simulink model "TV_2017"  (R2016a)
settings: Solver=FixedStepAuto  StartTime=0.0  StopTime=inf  FixedStep=0.001  RelTol=1e-3
PreLoadFcn:
  | TV_2017_parameters
values from neighbouring files (symbols this model uses):
  battery_voltage = single(530)    [HIL_parameters.m]    (also in HIL_parameters_2018.m; TV_2017_parameters.m; TV_2017_parameters_VD.m)
  car_params = Simulink_Car_params    [HIL_parameters.m]    (also in HIL_parameters_2018.m; TV_2017_parameters.m; TV_2017_parameters_VD.m)
  i_Diff = 16    [HIL_parameters.m]    (also in HIL_parameters_2018.m; TV_2017_parameters.m)
  Kp = 1    [HIL_parameters.m]    (also in HIL_parameters_2018.m; TV_2017_parameters.m; TV_2017_parameters_VD.m)
  motor_data = struct    [HIL_parameters.m]    (also in HIL_parameters_2018.m; TV_2017_parameters.m)
  powerLimitControl = Simulink_el    [HIL_parameters.m]    (also in HIL_parameters_2018.m; TV_2017_parameters.m; TV_2017_parameters_VD.m)
  settings = Simulink_Settings    [HIL_parameters.m]    (also in HIL_parameters_2018.m; TV_2017_parameters.m; TV_2017_parameters_VD.m)
  SpdC_BCC = 0    [HIL_parameters.m]    (also in HIL_parameters_2018.m; TV_2017_parameters.m; TV_2017_parameters_VD.m)
  Speed_Neg_sat = -21    [HIL_parameters.m]    (also in HIL_parameters_2018.m; TV_2017_parameters.m; TV_2017_parameters_VD.m)
  Speed_Pos_sat = 21    [HIL_parameters.m]    (also in HIL_parameters_2018.m; TV_2017_parameters.m; TV_2017_parameters_VD.m)
  SteeringAngleFL = [-23.80 -22.65 -21.50 -20.34 -19.18 -18.03 -16.86 -15.70 -14.53 -13.35 -12.18 -10.99 -9.80 -8.61 -7.40 -6.19 -4.97 -3.75 -2.51 -1.26 0 1.27 2.56 3.85 5.17 6.50 7.84 9.21 10.59 12.00 13.42 14.88 16.36 17.87 19.41 20.99 22.61 24.26 25.97 27.73 29.54]    [CarSetupAnalysis2018.m]    (also in HIL_parameters_2018.m; TV_2017_parameters.m; TV_2017_parameters_VD.m = [-24.129 -22.950 -21.772 -20.593 -19.413 -18.232 -17.050 -15)
  SteeringAngleFR = [-29.54 -27.73 -25.97 -24.26 -22.61 -20.99 -19.41 -17.87 -16.36 -14.88 -13.42 -12.00 -10.59 -9.21 -7.84 -6.50 -5.17 -3.85 -2.56 -1.27 0 1.26 2.51 3.75 4.97 6.19 7.40 8.61 9.80 10.99 12.18 13.35 14.53 15.70 16.86 18.03 19.18 20.34 21.50 22.65 23.80]    [CarSetupAnalysis2018.m]    (also in HIL_parameters_2018.m; TV_2017_parameters.m; TV_2017_parameters_VD.m = [-29.3050 -27.5340 -25.8140 -24.1410 -22.5110 -20.9180 -19.3)
  SteeringWhAngle = [-105 -99.75 -94.5 -89.25 -84 -78.75 -73.5 -68.25 -63 -57.75 -52.5 -47.25 -42 -36.75 -31.5 -26.25 -21.0 -15.75 -10.5 -5.25 0.0 5.25 10.50 15.75 21.00 26.25 31.50 36.75 42.00 47.25 52.50 57.75  63.00 68.25 73.50 78.75 84.00 89.25 94.50 99.75 105.00]    [TV_2017_parameters_VD.m]
  Tn_n = 0    [HIL_parameters.m]    (also in HIL_parameters_2018.m; TV_2017_parameters.m; TV_2017_parameters_VD.m)
  tractionControl = Simulink_tc    [HIL_parameters.m]    (also in HIL_parameters_2018.m; IterativeTractionControlTuning.m; TV_2017_parameters.m; TV_2017_parameters_VD.m)
  yawMomentGenerator = struct    [HIL_parameters.m]    (also in HIL_parameters_2018.m = Simulink_yawRate2; TV_2017_parameters.m = Simulink_yawRate2)
  yawRateControl = Simulink_yawRate    [HIL_parameters.m]    (also in HIL_parameters_2018.m; TV_2017_parameters.m; TV_2017_parameters_VD.m)
undefined symbols (not defined in the file or in its folder): DiscIntNeverNeededParam, magnitude, speedEstimation, TC_Decr_Gas, TC_Derivative, TC_Incr_Gas, TC_On, TC_Relay_Off, TC_Relay_On
libraries: CarMaker4SL x350, simulink_extras x63, simulink x37, dspfdesign x2
(part 6 of 14)

== system TV_2017/CarMaker/Estimations/Fz_estimators/Fz_Estimation ==
  sensors : Inport
  1st_deriv : Subsystem
  2nd_deriv : Subsystem
  Bus Selector : BusSelector  OutputSignals=damper_rate_FL,damper_rate_FR,damper_rate_RL,damper_rate_RR
  Bus Selector1 : BusSelector  OutputSignals=FL,FR,RL,RR
  DamperRateLookup : Lookup_n-D  NumberOfTableDimensions=1  BreakpointsForDimension1=car_params.damper_table_breakpoint;  Table=car_params.damper_pull_push_values_front;  ExtrapMethod=Clip  UseLastTableValue=on  InternalRulePriority=Speed  RndMeth=Simplest  InputSameDT=on
  DamperRateLookup1 : Lookup_n-D  NumberOfTableDimensions=1  BreakpointsForDimension1=car_params.damper_table_breakpoint;  Table=car_params.damper_pull_push_values_front;  ExtrapMethod=Clip  UseLastTableValue=on  InternalRulePriority=Speed  RndMeth=Simplest  InputSameDT=on
  DamperRateLookup2 : Lookup_n-D  NumberOfTableDimensions=1  BreakpointsForDimension1=car_params.damper_table_breakpoint;  Table=car_params.damper_pull_push_values_rear;  ExtrapMethod=Clip  UseLastTableValue=on  InternalRulePriority=Speed  RndMeth=Simplest  InputSameDT=on
  DamperRateLookup3 : Lookup_n-D  NumberOfTableDimensions=1  BreakpointsForDimension1=car_params.damper_table_breakpoint;  Table=car_params.damper_pull_push_values_rear;  ExtrapMethod=Clip  UseLastTableValue=on  InternalRulePriority=Speed  RndMeth=Simplest  InputSameDT=on
  FZ_etsimate : Scope  NumInputPorts=4
  FzEstDamper : MATLAB Function  TreatAsAtomicUnit=on
  Scope2 : Scope  NumInputPorts=4
  Sum : Sum  Inputs=|++++
  Sum_FZ : Scope
  alfa_r_scope : Scope
  Fz_est : Outport
  alfa_r : Outport  Port=2
  wires:
  sensors/1 -> FzEstDamper/1(sensors), Bus Selector/1
  Bus Selector/1 -> DamperRateLookup/1  "<damper_rate_FL>"
  Bus Selector/2 -> DamperRateLookup1/1  "<damper_rate_FR>"
  Bus Selector/3 -> DamperRateLookup2/1  "<damper_rate_RL>"
  Bus Selector/4 -> DamperRateLookup3/1  "<damper_rate_RR>"
  FzEstDamper/2(alfa_r) -> alfa_r_scope/1, alfa_r/1
  Bus Selector1/2 -> Sum/3, FZ_etsimate/2  "<FR>"
  Bus Selector1/1 -> Sum/4, FZ_etsimate/1  "<FL>"
  Bus Selector1/3 -> Sum/2, FZ_etsimate/3  "<RL>"
  Bus Selector1/4 -> FZ_etsimate/4, Sum/1  "<RR>"
  FzEstDamper/1(Fz_damper_est) -> Bus Selector1/1, Fz_est/1
  DamperRateLookup1/1 -> Scope2/2, FzEstDamper/3(Fz_damp_FR)  "<FR>"
  DamperRateLookup/1 -> Scope2/1, FzEstDamper/2(Fz_damp_FL)  "<FL>"
  DamperRateLookup2/1 -> Scope2/3, FzEstDamper/4(Fz_damp_RL)  "<RL>"
  DamperRateLookup3/1 -> Scope2/4, FzEstDamper/5(Fz_damp_RR)  "<RR>"
  Sum/1 -> Sum_FZ/1

== system TV_2017/CarMaker/Estimations/Fz_estimators/Fz_Estimation_acceleration based ==
  sensors : Inport
  Bus Selector1 : BusSelector  OutputSignals=FL,FR,RL,RR
  Bus Selector2 : BusSelector  OutputSignals=Input_throttle,Input_brake,KERS_pos
  FZ_etsimate_acceleration : Scope  NumInputPorts=4
  Fz_acc_est : MATLAB Function  TreatAsAtomicUnit=on
  Lowpass Filter : dspfdesign/Lowpass Filter  FilterType=FIR  DesignForMinimumOrder=on  FilterOrder=50  PassbandFrequency=4  StopbandFrequency=15  PassbandRipple=0.1  StopbandAttenuation=80  InheritSampleRate=on  SampleRate=100  roundingMode=Floor  coeffsDataTypeStr=fixdt(1,16)  SimulateUsing=Interpreted execution
  Lowpass Filter1 : dspfdesign/Lowpass Filter  FilterType=FIR  DesignForMinimumOrder=on  FilterOrder=50  PassbandFrequency=4  StopbandFrequency=15  PassbandRipple=0.1  StopbandAttenuation=80  InheritSampleRate=on  SampleRate=100  roundingMode=Floor  coeffsDataTypeStr=fixdt(1,16)  SimulateUsing=Code generation
  alfa_r_acc : Scope  NumInputPorts=2
  alfa_r_acc_tps_bps_kers : Scope  NumInputPorts=4
  filtervsUnfilter : Scope  NumInputPorts=2
  "Fz_acc " : Outport
  "alfa_r_acc " : Outport  Port=2
  wires:
  sensors/1 -> Bus Selector2/1, Fz_acc_est/1(sensors)
  Bus Selector1/2 -> FZ_etsimate_acceleration/2  "<FR>"
  Bus Selector1/1 -> Lowpass Filter/1, filtervsUnfilter/2, FZ_etsimate_acceleration/1  "<FL>"
  Bus Selector1/3 -> FZ_etsimate_acceleration/3  "<RL>"
  Bus Selector1/4 -> FZ_etsimate_acceleration/4  "<RR>"
  Fz_acc_est/1(Fz_acc_est) -> "Fz_acc "/1, Bus Selector1/1
  Lowpass Filter/1 -> filtervsUnfilter/1
  Lowpass Filter1/1 -> alfa_r_acc/1
  Fz_acc_est/2(alfa_r_acc) -> alfa_r_acc_tps_bps_kers/1, "alfa_r_acc "/1, alfa_r_acc/2, Lowpass Filter1/1
  Bus Selector2/1 -> alfa_r_acc_tps_bps_kers/2  "<Input_throttle>"
  Bus Selector2/2 -> alfa_r_acc_tps_bps_kers/3  "<Input_brake>"
  Bus Selector2/3 -> alfa_r_acc_tps_bps_kers/4  "<KERS_pos>"

== system TV_2017/CarMaker/Estimations/Subsystem/SA calculation ==
  sensor : Inport
  Bus Selector2 : BusSelector  OutputSignals=steering_wheel_angle
  Degrees to Radians : simulink_extras/Transformations/Degrees to Radians
  Degrees to Radians1 : simulink_extras/Transformations/Degrees to Radians
  FL steer ang lookup deg : Lookup_n-D  NumberOfTableDimensions=1  BreakpointsForDimension1=SteeringAngleFL  Table=SteeringAngleFL  ExtrapMethod=Clip  UseLastTableValue=on  InternalRulePriority=Speed  RndMeth=Simplest  InputSameDT=on
  FR steer ang lookup deg : Lookup_n-D  NumberOfTableDimensions=1  BreakpointsForDimension1=SteeringAngleFR  Table=SteeringAngleFR  ExtrapMethod=Clip  UseLastTableValue=on  InternalRulePriority=Speed  RndMeth=Simplest  InputSameDT=on
  Radians to Degrees1 : simulink_extras/Transformations/Radians to Degrees
  Slip angle calc : MATLAB Function  Commented=on  TreatAsAtomicUnit=on
  Slip angle calc1 : MATLAB Function  TreatAsAtomicUnit=on
  SA : Outport
  wires:
  Radians to Degrees1/1 -> FL steer ang lookup deg/1, FR steer ang lookup deg/1
  Degrees to Radians1/1 -> Slip angle calc1/2(wheel_ang_right)
  Slip angle calc1/1(SA) -> SA/1
  FR steer ang lookup deg/1 -> Degrees to Radians1/1
  sensor/1 -> Slip angle calc1/3(sensor), Bus Selector2/1
  FL steer ang lookup deg/1 -> Degrees to Radians/1
  Bus Selector2/1 -> Radians to Degrees1/1  "<steering_wheel_angle>"
  Degrees to Radians/1 -> Slip angle calc1/1(wheel_ang_left)

== system TV_2017/CarMaker/Estimations/Subsystem/SR_Calculation ==
  v_x : Inport
  whl_v : Inport  Port=2
  sensorInput : Inport  Port=3
  Slip ratio : MATLAB Function  TreatAsAtomicUnit=on
  SR : Outport
  wires:
  v_x/1 -> Slip ratio/1(V_x)
  Slip ratio/1(SR) -> SR/1
  whl_v/1 -> Slip ratio/2(whl_v)
  sensorInput/1 -> Slip ratio/3(sensor)

== system TV_2017/CarMaker/Estimations/Subsystem/Slip_Detection ==
  sensor : Inport
  SR : Inport  Port=2
  Memory : Memory  InheritSampleTime=on
  Slip Detection : MATLAB Function  TreatAsAtomicUnit=on
  slip : Outport
  wires:
  Slip Detection/1(slip) -> Memory/1, slip/1
  SR/1 -> Slip Detection/1(SR)
  sensor/1 -> Slip Detection/2(sensors)
  Memory/1 -> Slip Detection/3(slip_prev)

== system TV_2017/CarMaker/IPG Vehicle3/Brake/CreateBus Vhcl.Wheel.PT ==
  In : Inport
  BusCreator1 : BusCreator  Inputs=20
  Demux1 : Demux  Outputs=20
  Out : Outport
  wires:
  Demux1/20 -> BusCreator1/20  "Vhcl Trq_DriveSrc_trg d3"
  Demux1/19 -> BusCreator1/19  "Vhcl Trq_DriveSrc_trg d2"
  Demux1/18 -> BusCreator1/18  "Vhcl Trq_DriveSrc_trg d1"
  Demux1/17 -> BusCreator1/17  "Vhcl Trq_DriveSrc_trg d0"
  Demux1/16 -> BusCreator1/16  "Vhcl Wheel RR WhlBearing"
  Demux1/15 -> BusCreator1/15  "Vhcl Wheel RR Trq_T2W"
  Demux1/14 -> BusCreator1/14  "Vhcl Wheel RR Trq_BrakeReg_trg"
  Demux1/13 -> BusCreator1/13  "Vhcl Wheel RR Trq_Brake"
  Demux1/12 -> BusCreator1/12  "Vhcl Wheel RL WhlBearing"
  Demux1/11 -> BusCreator1/11  "Vhcl Wheel RL Trq_T2W"
  Demux1/10 -> BusCreator1/10  "Vhcl Wheel RL Trq_BrakeReg_trg"
  Demux1/9 -> BusCreator1/9  "Vhcl Wheel RL Trq_Brake"
  Demux1/8 -> BusCreator1/8  "Vhcl Wheel FR WhlBearing"
  Demux1/7 -> BusCreator1/7  "Vhcl Wheel FR Trq_T2W"
  Demux1/6 -> BusCreator1/6  "Vhcl Wheel FR Trq_BrakeReg_trg"
  Demux1/5 -> BusCreator1/5  "Vhcl Wheel FR Trq_Brake"
  Demux1/4 -> BusCreator1/4  "Vhcl Wheel FL WhlBearing"
  Demux1/3 -> BusCreator1/3  "Vhcl Wheel FL Trq_T2W"
  Demux1/2 -> BusCreator1/2  "Vhcl Wheel FL Trq_BrakeReg_trg"
  Demux1/1 -> BusCreator1/1  "Vhcl Wheel FL Trq_Brake"
  BusCreator1/1 -> Out/1
  In/1 -> Demux1/1

== system TV_2017/CarMaker/IPG Vehicle3/CarAndTrailer/CarAndTrailerUpd ==
  Sync_In : Inport
  Vhcl.Steering : Inport  Port=2
  Vhcl.Motion : Inport  Port=3
  Vhcl.PoI : Inport  Port=4
  Vhcl.Wheel.FL : Inport  Port=5
  Vhcl.Wheel.FR : Inport  Port=6
  Vhcl.Wheel.RL : Inport  Port=7
  Vhcl.Wheel.RR : Inport  Port=8
  Car.Hitch.FrcTrq : Inport  Port=9
  Vhcl.Fr1A : Inport  Port=10
  CarAndTrailerUpd : S-Function  FunctionName=CM_Sfun  Parameters='CarAndTrUpd'  SFunctionDeploymentMode=off  EnableBusSupport=off
  CreateBus Brake.IF.In : Subsystem
  Sync_Out : Outport
  Brake.IF.In : Outport  Port=2
  wires:
  Vhcl.Fr1A/1 -> CarAndTrailerUpd/10  "user vehicle only"
  Vhcl.Steering/1 -> CarAndTrailerUpd/2
  Vhcl.Motion/1 -> CarAndTrailerUpd/3
  Vhcl.PoI/1 -> CarAndTrailerUpd/4
  Vhcl.Wheel.FL/1 -> CarAndTrailerUpd/5
  Vhcl.Wheel.FR/1 -> CarAndTrailerUpd/6
  Car.Hitch.FrcTrq/1 -> CarAndTrailerUpd/9
  Vhcl.Wheel.RR/1 -> CarAndTrailerUpd/8
  Vhcl.Wheel.RL/1 -> CarAndTrailerUpd/7
  CarAndTrailerUpd/2 -> CreateBus Brake.IF.In/1(In)
  CreateBus Brake.IF.In/1(Out) -> Brake.IF.In/1
  CarAndTrailerUpd/1 -> Sync_Out/1
  Sync_In/1 -> CarAndTrailerUpd/1

== system TV_2017/CarMaker/IPG Vehicle3/CarAndTrailer/Forces ==
  Sync_In : Inport
  TireFL_In : Inport  Port=2
  TireFR_In : Inport  Port=3
  TireRL_In : Inport  Port=4
  TireRR_In : Inport  Port=5
  lSpring : Inport  Port=6
  vDamp : Inport  Port=7
  lStabi : Inport  Port=8
  lBuf : Inport  Port=9
  External Suspension Forces : Subsystem
  Tires : Subsystem
  Vehicle Forces : Subsystem
  Sync_Out : Outport
  Car.Virtual : Outport  Port=2
  Car.Aero : Outport  Port=3
  Car.Load : Outport  Port=4
  TireFL_Out : Outport  Port=5
  TireFR_Out : Outport  Port=6
  TireRL_Out : Outport  Port=7
  TireRR_Out : Outport  Port=8
  FSpring : Outport  Port=9
  FDamp : Outport  Port=10
  FStabi : Outport  Port=11
  FBuf : Outport  Port=12
  wires:
  lBuf/1 -> External Suspension Forces/5(lBuf)
  lStabi/1 -> External Suspension Forces/4(lStabi)
  vDamp/1 -> External Suspension Forces/3(vDamp)
  Tires/4(TireRR_Out) -> TireRR_Out/1
  Tires/3(TireRL_Out) -> TireRL_Out/1
  Tires/2(TireFR_Out) -> TireFR_Out/1
  Tires/1(TireFL_Out) -> TireFL_Out/1
  TireRR_In/1 -> Tires/5(TireRR_In)
  TireRL_In/1 -> Tires/4(TireRL_In)
  TireFR_In/1 -> Tires/3(TireFR_In)
  TireFL_In/1 -> Tires/2(TireFL_In)
  External Suspension Forces/4(FBuf) -> FBuf/1
  Sync_In/1 -> External Suspension Forces/1(Sync_In), Tires/1(Sync_In), Vehicle Forces/1(Sync_In)
  Vehicle Forces/1(Sync_Out) -> Sync_Out/1
  Vehicle Forces/2(Car.Virtual) -> Car.Virtual/1
  Vehicle Forces/3(Car.Aero) -> Car.Aero/1
  Vehicle Forces/4(Car.Load) -> Car.Load/1
  lSpring/1 -> External Suspension Forces/2(lSpring)
  External Suspension Forces/2(FDamp) -> FDamp/1
  External Suspension Forces/3(FStabi) -> FStabi/1
  External Suspension Forces/1(FSpring) -> FSpring/1

== system TV_2017/CarMaker/IPG Vehicle3/CarAndTrailer/Kinematics ==
  Sync_In : Inport
  Steer.IF : Inport  Port=2
  Kinematics : S-Function  FunctionName=CM_Sfun  Parameters='Kinematics'  SFunctionDeploymentMode=off  EnableBusSupport=off
  Sync_Out : Outport
  TireFL_In : Outport  Port=2
  TireFR_In : Outport  Port=3
  TireRL_In : Outport  Port=4
  TireRR_In : Outport  Port=5
  lSpring : Outport  Port=6
  vDamp : Outport  Port=7
  lStabi : Outport  Port=8
  lBuf : Outport  Port=9
  wires:
  Kinematics/9 -> lBuf/1
  Kinematics/8 -> lStabi/1
  Kinematics/2 -> TireFL_In/1
  Kinematics/3 -> TireFR_In/1
  Kinematics/4 -> TireRL_In/1
  Kinematics/5 -> TireRR_In/1
  Kinematics/6 -> lSpring/1
  Kinematics/7 -> vDamp/1
  Sync_In/1 -> Kinematics/1
  Kinematics/1 -> Sync_Out/1
  Steer.IF/1 -> Kinematics/2

== system TV_2017/CarMaker/IPG Vehicle3/CarAndTrailer/Kinetics ==
  Sync_In : Inport
  Car.Virtual : Inport  Port=2
  Car.Aero : Inport  Port=3
  Car.Load : Inport  Port=4
  TireFL.Out : Inport  Port=5
  TireFR.Out : Inport  Port=6
  TireRL.Out : Inport  Port=7
  TireRR.Out : Inport  Port=8
  FSpring : Inport  Port=9
  FDamp : Inport  Port=10
  FStabi : Inport  Port=11
  FBuf : Inport  Port=12
  Bus Creator : BusCreator  Inputs=4
  Bus Creator1 : BusCreator  Inputs=12
  Bus Creator2 : BusCreator  Inputs=6
  Bus Creator3 : BusCreator  Inputs=6
  Bus Creator4 : BusCreator  Inputs=4
  Demux : Demux  Outputs=12
  Demux1 : Demux  Outputs=6
  Demux2 : Demux  Outputs=6
  Demux3 : Demux
  Demux4 : Demux
  Kinetics : S-Function  FunctionName=CM_Sfun  Parameters='Kinetics'  SFunctionDeploymentMode=off  EnableBusSupport=off
  Sync_Out : Outport
  Trailer.Load : Outport  Port=2
  Car.Hitch : Outport  Port=3
  Car.Fr1 : Outport  Port=4
  Car.Trq_T2W : Outport  Port=5
  WheelCarrier.Misc : Outport  Port=6
  wires:
  FBuf/1 -> Kinetics/12
  Sync_In/1 -> Kinetics/1
  Kinetics/1 -> Sync_Out/1
  Car.Aero/1 -> Kinetics/3
  Car.Virtual/1 -> Kinetics/2
  Bus Creator1/1 -> Trailer.Load/1
  Demux/1 -> Bus Creator1/1  "Trailer Load_0 mass"
  Demux/2 -> Bus Creator1/2  "Trailer Load_0 tx"
  Demux/3 -> Bus Creator1/3  "Trailer Load_0 ty"
  Demux/4 -> Bus Creator1/4  "Trailer Load_0 tz"
  Kinetics/2 -> Demux/1
  Demux/5 -> Bus Creator1/5  "Trailer Load_1 mass"
  Demux/6 -> Bus Creator1/6  "Trailer Load_1 tx"
  Demux/7 -> Bus Creator1/7  "Trailer Load_1 ty"
  Demux/8 -> Bus Creator1/8  "Trailer Load_1 tz"
  Demux/9 -> Bus Creator1/9  "Trailer Load_2 mass"
  Demux/10 -> Bus Creator1/10  "Trailer Load_2 tx"
  Demux/11 -> Bus Creator1/11  "Trailer Load_2 ty"
  Demux/12 -> Bus Creator1/12  "Trailer Load_2 tz"
  Demux1/1 -> Bus Creator2/1  "Car Hitch tx"
  Demux1/2 -> Bus Creator2/2  "Car Hitch ty"
  Demux1/3 -> Bus Creator2/3  "Car Hitch tz"
  Demux1/4 -> Bus Creator2/4  "Car Hitch vx"
  Demux1/5 -> Bus Creator2/5  "Car Hitch vy"
  Demux1/6 -> Bus Creator2/6  "Car Hitch vz"
  Kinetics/3 -> Demux1/1
  Bus Creator2/1 -> Car.Hitch/1
  Demux2/1 -> Bus Creator3/1  "Car Fr1 rx"
  Demux2/2 -> Bus Creator3/2  "Car Fr1 ry"
  Demux2/3 -> Bus Creator3/3  "Car Fr1 rz"
  Demux2/4 -> Bus Creator3/4  "Car Fr1 rvx"
  Demux2/5 -> Bus Creator3/5  "Car Fr1 rvy"
  Demux2/6 -> Bus Creator3/6  "Car Fr1 rvz"
  Bus Creator3/1 -> Car.Fr1/1
  Kinetics/4 -> Demux2/1
  Car.Load/1 -> Kinetics/4
  Demux3/1 -> Bus Creator4/1  "car Susp FL GenInert2"
  Demux3/2 -> Bus Creator4/2  "car Susp FR GenInert2"
  Demux3/3 -> Bus Creator4/3  "car Susp FL GenFrc2"
  Demux3/4 -> Bus Creator4/4  "car Susp FR GenFrc2"
  Bus Creator4/1 -> WheelCarrier.Misc/1
  Bus Creator/1 -> Car.Trq_T2W/1
  Demux4/4 -> Bus Creator/4  "Car Trq_T2WRR"
  Demux4/3 -> Bus Creator/3  "Car Trq_T2WRL"
  Demux4/2 -> Bus Creator/2  "Car Trq_T2WFR"
  Demux4/1 -> Bus Creator/1  "Car Trq_T2WFL"
  TireFL.Out/1 -> Kinetics/5
  TireFR.Out/1 -> Kinetics/6
  TireRL.Out/1 -> Kinetics/7
  TireRR.Out/1 -> Kinetics/8
  FSpring/1 -> Kinetics/9
  FDamp/1 -> Kinetics/10
  FStabi/1 -> Kinetics/11
  Kinetics/6 -> Demux3/1
  Kinetics/5 -> Demux4/1

== system TV_2017/CarMaker/IPG Vehicle3/CarAndTrailer/Steering ==
  note: When replacing the entire steering system,
      | be sure to add '-disablesteering' to the command line arguments
      | in the CarMaker Model Configuration block.
  Sync_In : Inport
  VhclCtrl.Steering : Inport  Port=2
  Bus Creator1 : BusCreator  Inputs=16
  Bus Creator2 : BusCreator  Inputs=5
  Demux : Demux  Outputs=21
  Steering : S-Function  FunctionName=CM_Sfun  Parameters='Steering'  SFunctionDeploymentMode=off  EnableBusSupport=off
  Terminator : Terminator
  Sync_Out : Outport
  Steer.IF : Outport  Port=2
  wires:
  Demux/21 -> Bus Creator2/5  "Steering IF R Inert"
  Demux/20 -> Bus Creator2/4  "Steering IF R Frc"
  Demux/19 -> Bus Creator2/3  "Steering IF L Inert"
  Demux/18 -> Bus Creator2/2  "Steering IF L Frc"
  Demux/17 -> Bus Creator2/1  "Steering IF SteerByTrq"
  Demux/16 -> Bus Creator1/16  "Steering IF R iSteer2q"
  Demux/15 -> Bus Creator1/15  "Steering IF R qpp"
  Demux/14 -> Bus Creator1/14  "Steering IF R qp"
  Demux/13 -> Bus Creator1/13  "Steering IF R q"
  Demux/12 -> Bus Creator1/12  "Steering IF L iSteer2q"
  Demux/11 -> Bus Creator1/11  "Steering IF L qpp"
  Demux/10 -> Bus Creator1/10  "Steering IF L qp"
  Demux/9 -> Bus Creator1/9  "Steering IF L q"
  Demux/8 -> Bus Creator1/8  "Steering IF AssistTrqPin"
  Demux/7 -> Bus Creator1/7  "Steering IF AssistTrqCol"
  Demux/6 -> Bus Creator1/6  "Steering IF AssistFrc"
  Demux/5 -> Bus Creator1/5  "Steering IF TrqStatic"
  Demux/4 -> Bus Creator1/4  "Steering IF Trq"
  Demux/3 -> Bus Creator1/3  "Steering IF AngAcc"
  Demux/2 -> Bus Creator1/2  "Steering IF AngVel"
  Demux/1 -> Bus Creator1/1  "Steering IF Ang"
  Bus Creator1/1 -> Steer.IF/1
  Steering/2 -> Demux/1
  Bus Creator2/1 -> Terminator/1  "Steer IF (in)"
  VhclCtrl.Steering/1 -> Steering/2
  Steering/1 -> Sync_Out/1
  Sync_In/1 -> Steering/1

== system TV_2017/CarMaker/IPG Vehicle3/CarAndTrailer/Trailer ==
  Sync_In : Inport
  Trailer.Load : Inport  Port=2
  Car.Hitch : Inport  Port=3
  Car.Fr1 : Inport  Port=4
  Car.Trq_T2W : Inport  Port=5
  WheelCarrier.Misc : Inport  Port=6
  CreateBus Car.Hitch.FrcTrq : Subsystem
  CreateBus Vhcl.Motion : Subsystem
  CreateBus Vhcl.PoI : Subsystem
  CreateBus Vhcl.Steering : Subsystem
  CreateBus Vhcl.Wheel.FL : Subsystem
  CreateBus Vhcl.Wheel.FR : Subsystem
  CreateBus Vhcl.Wheel.RL : Subsystem
  CreateBus Vhcl.Wheel.RR : Subsystem
  Trailer : S-Function  FunctionName=CM_Sfun  Parameters='Trailer'  SFunctionDeploymentMode=off  EnableBusSupport=off
  Sync_Out : Outport
  Vhcl.Steering : Outport  Port=2
  Vhcl.Motion : Outport  Port=3
  Vhcl.PoI : Outport  Port=4
  Vhcl.Wheel.FL : Outport  Port=5
  Vhcl.Wheel.FR : Outport  Port=6
  Vhcl.Wheel.RL : Outport  Port=7
  Vhcl.Wheel.RR : Outport  Port=8
  Car.Hitch.FrcTrq : Outport  Port=9
  wires:
  Trailer/2 -> CreateBus Vhcl.Steering/1(In1)
  CreateBus Vhcl.Steering/1(Out1) -> Vhcl.Steering/1  "Vhcl.Steering"
  Trailer/3 -> CreateBus Vhcl.Motion/1(In1)
  Trailer/4 -> CreateBus Vhcl.PoI/1(In1)
  Trailer/5 -> CreateBus Vhcl.Wheel.FL/1(In1)
  Trailer/6 -> CreateBus Vhcl.Wheel.FR/1(In1)
  Trailer/7 -> CreateBus Vhcl.Wheel.RL/1(In1)
  Trailer/9 -> CreateBus Car.Hitch.FrcTrq/1(In1)
  Trailer/8 -> CreateBus Vhcl.Wheel.RR/1(In1)
  CreateBus Vhcl.Wheel.RR/1(Out1) -> Vhcl.Wheel.RR/1  "Vhcl.Wheel.RR"
  CreateBus Vhcl.Wheel.RL/1(Out1) -> Vhcl.Wheel.RL/1  "Vhcl.Wheel.RL"
  CreateBus Vhcl.Wheel.FR/1(Out1) -> Vhcl.Wheel.FR/1  "Vhcl.Wheel.FR"
  CreateBus Vhcl.Wheel.FL/1(Out1) -> Vhcl.Wheel.FL/1  "Vhcl.Wheel.FL"
  CreateBus Vhcl.PoI/1(Out1) -> Vhcl.PoI/1  "Vhcl.PoI"
  CreateBus Vhcl.Motion/1(Out1) -> Vhcl.Motion/1  "Vhcl.Motion"
  Car.Trq_T2W/1 -> Trailer/5
  WheelCarrier.Misc/1 -> Trailer/6
  CreateBus Car.Hitch.FrcTrq/1(Out1) -> Car.Hitch.FrcTrq/1  "Car.Hitch.FrcTrq"
  Car.Fr1/1 -> Trailer/4
  Car.Hitch/1 -> Trailer/3
  Trailer.Load/1 -> Trailer/2
  Trailer/1 -> Sync_Out/1
  Sync_In/1 -> Trailer/1

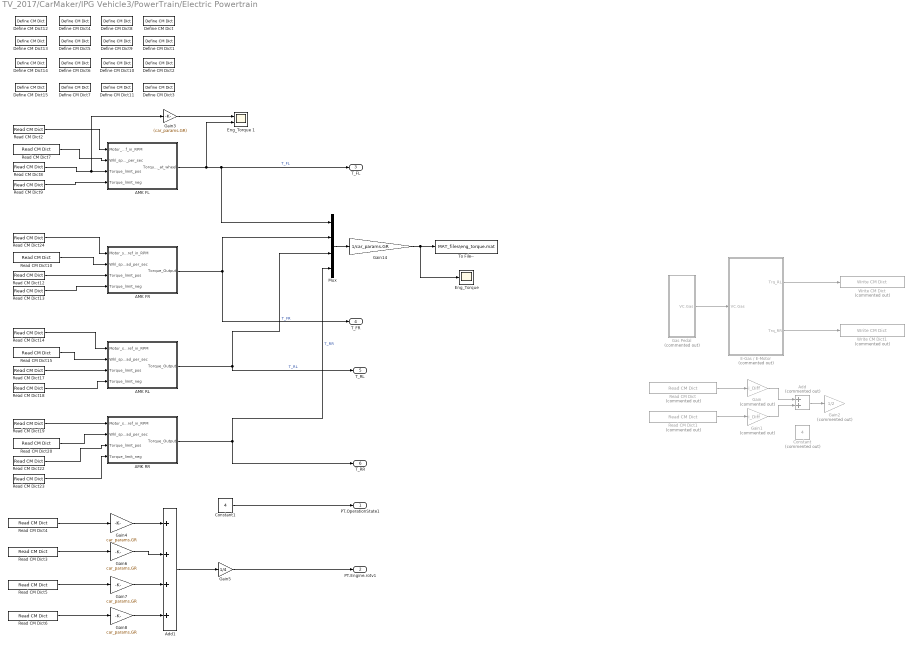
== system TV_2017/CarMaker/IPG Vehicle3/PowerTrain/Electric Powertrain ==
  AMK FL : Subsystem
  AMK FR : Subsystem
  AMK RL : Subsystem
  AMK RR : Subsystem
  Add : Sum  Commented=on
  Add1 : Sum  Inputs=++++
  Constant : Constant  Commented=on  Value=4
  Constant1 : Constant  Value=4
  Define CM Dict : CarMaker4SL/Define CM Dict  xname=T_req_RL  xmono=off  xtype=Double4  xdvaplace=None  xnstates=0  xfirststate=0  xinitial=0
  Define CM Dict1 : CarMaker4SL/Define CM Dict  xname=T_req_RR  xmono=off  xtype=Double4  xdvaplace=None  xnstates=0  xfirststate=0  xinitial=0
  Define CM Dict10 : CarMaker4SL/Define CM Dict  xname=Tlim_neg_RL  xmono=off  xtype=Double4  xdvaplace=None  xnstates=0  xfirststate=0  xinitial=0
  Define CM Dict11 : CarMaker4SL/Define CM Dict  xname=Tlim_neg_RR  xmono=off  xtype=Double4  xdvaplace=None  xnstates=0  xfirststate=0  xinitial=0
  Define CM Dict12 : CarMaker4SL/Define CM Dict  xname=w_set_FL  xmono=off  xtype=Double4  xdvaplace=None  xnstates=0  xfirststate=0  xinitial=0
  Define CM Dict13 : CarMaker4SL/Define CM Dict  xname=w_set_FR  xmono=off  xtype=Double4  xdvaplace=None  xnstates=0  xfirststate=0  xinitial=0
  Define CM Dict14 : CarMaker4SL/Define CM Dict  xname=w_set_RL  xmono=off  xtype=Double4  xdvaplace=None  xnstates=0  xfirststate=0  xinitial=0
  Define CM Dict15 : CarMaker4SL/Define CM Dict  xname=w_set_RR  xmono=off  xtype=Double4  xdvaplace=None  xnstates=0  xfirststate=0  xinitial=0
  Define CM Dict2 : CarMaker4SL/Define CM Dict  xname=T_req_FL  xmono=off  xtype=Double4  xdvaplace=None  xnstates=0  xfirststate=0  xinitial=0
  Define CM Dict3 : CarMaker4SL/Define CM Dict  xname=T_req_FR  xmono=off  xtype=Double4  xdvaplace=None  xnstates=0  xfirststate=0  xinitial=0
  Define CM Dict4 : CarMaker4SL/Define CM Dict  xname=Tlim_pos_FL  xmono=off  xtype=Double4  xdvaplace=None  xnstates=0  xfirststate=0  xinitial=0
  Define CM Dict5 : CarMaker4SL/Define CM Dict  xname=Tlim_pos_FR  xmono=off  xtype=Double4  xdvaplace=None  xnstates=0  xfirststate=0  xinitial=0
  Define CM Dict6 : CarMaker4SL/Define CM Dict  xname=Tlim_pos_RL  xmono=off  xtype=Double4  xdvaplace=None  xnstates=0  xfirststate=0  xinitial=0
  Define CM Dict7 : CarMaker4SL/Define CM Dict  xname=Tlim_pos_RR  xmono=off  xtype=Double4  xdvaplace=None  xnstates=0  xfirststate=0  xinitial=0
  Define CM Dict8 : CarMaker4SL/Define CM Dict  xname=Tlim_neg_FL  xmono=off  xtype=Double4  xdvaplace=None  xnstates=0  xfirststate=0  xinitial=0
  Define CM Dict9 : CarMaker4SL/Define CM Dict  xname=Tlim_neg_FR  xmono=off  xtype=Double4  xdvaplace=None  xnstates=0  xfirststate=0  xinitial=0
  E-Gas / E-Motor : Subsystem  Commented=on
  "Eng_Torque " : Scope
  Eng_Torque 1 : Scope  NumInputPorts=2
  Gain : Gain  Commented=on  Gain=i_Diff
  Gain1 : Gain  Commented=on  Gain=i_Diff
  Gain14 : Gain  Gain=1/car_params.GR
  Gain2 : Gain  Commented=on  Gain=1/2
  Gain3 : Gain  Gain=(car_params.GR)
  Gain{4,6..8} (4 alike) : Gain  Gain=car_params.GR
  Gain5 : Gain  Gain=1/4
  Gas Pedal : Subsystem  Commented=on
  Mux : Mux
  Read CM Dict : CarMaker4SL/Read CM Dict  Commented=on  xname=Car.WheelSpd_RL  xsync=off
  Read CM Dict1 : CarMaker4SL/Read CM Dict  Commented=on  xname=Car.WheelSpd_RR  xsync=off
  Read CM Dict10 : CarMaker4SL/Read CM Dict  xname=Car.WheelSpd_FR  xsync=off
  Read CM Dict12 : CarMaker4SL/Read CM Dict  xname=Tlim_pos_FR  xsync=off
  Read CM Dict13 : CarMaker4SL/Read CM Dict  xname=Tlim_neg_FR  xsync=off
  Read CM Dict14 : CarMaker4SL/Read CM Dict  xname=w_set_RL  xsync=off
  Read CM Dict15 : CarMaker4SL/Read CM Dict  xname=Car.WheelSpd_RL  xsync=off
  Read CM Dict17 : CarMaker4SL/Read CM Dict  xname=Tlim_pos_RL  xsync=off
  Read CM Dict18 : CarMaker4SL/Read CM Dict  xname=Tlim_neg_RL  xsync=off
  Read CM Dict19 : CarMaker4SL/Read CM Dict  xname=w_set_RR  xsync=off
  Read CM Dict2 : CarMaker4SL/Read CM Dict  xname=w_set_FL  xsync=off
  Read CM Dict20 : CarMaker4SL/Read CM Dict  xname=Car.WheelSpd_RR  xsync=off
  Read CM Dict22 : CarMaker4SL/Read CM Dict  xname=Tlim_pos_RR  xsync=off
  Read CM Dict23 : CarMaker4SL/Read CM Dict  xname=Tlim_neg_RR  xsync=off
  Read CM Dict24 : CarMaker4SL/Read CM Dict  xname=w_set_FR  xsync=off
  Read CM Dict3 : CarMaker4SL/Read CM Dict  xname=Car.WheelSpd_RR  xsync=off
  Read CM Dict4 : CarMaker4SL/Read CM Dict  xname=Car.WheelSpd_RL  xsync=off
  Read CM Dict5 : CarMaker4SL/Read CM Dict  xname=Car.WheelSpd_FR  xsync=off
  Read CM Dict6 : CarMaker4SL/Read CM Dict  xname=Car.WheelSpd_FL  xsync=off
  Read CM Dict7 : CarMaker4SL/Read CM Dict  xname=Car.WheelSpd_FL  xsync=off
  Read CM Dict8 : CarMaker4SL/Read CM Dict  xname=Tlim_pos_FL  xsync=off
  Read CM Dict9 : CarMaker4SL/Read CM Dict  xname=Tlim_neg_FL  xsync=off
  To File-- : ToFile  Filename=MAT_files\eng_torque.mat  MatrixName=torques  SaveFormat=Timeseries
  Write CM Dict : CarMaker4SL/Write CM Dict  Commented=on  xname=PT.WRL.Trq_Drive  xsync=off
  Write CM Dict1 : CarMaker4SL/Write CM Dict  Commented=on  xname=PT.WRR.Trq_Drive  xsync=off
  PT.OperationState1 : Outport
  PT.Engine.rotv1 : Outport  Port=2
  T_FL : Outport  Port=3
  T_FR : Outport  Port=4
  T_RL : Outport  Port=5
  T_RR : Outport  Port=6
  wires:
  Gas Pedal/1(VC.Gas) -> E-Gas / E-Motor/1(VC.Gas)
  E-Gas / E-Motor/1(Trq_RL) -> Write CM Dict/1
  E-Gas / E-Motor/2(Trq_RR) -> Write CM Dict1/1
  Read CM Dict1/1 -> Gain1/1
  Read CM Dict/1 -> Gain/1
  Gain/1 -> Add/1
  Gain1/1 -> Add/2
  Add/1 -> Gain2/1
  Constant1/1 -> PT.OperationState1/1
  Gain4/1 -> Add1/1
  Gain6/1 -> Add1/2
  Add1/1 -> Gain5/1
  Gain5/1 -> PT.Engine.rotv1/1
  Gain7/1 -> Add1/3
  Gain8/1 -> Add1/4
  Read CM Dict7/1 -> AMK FL/2(Whl_speed_rad_per_sec)
  Read CM Dict9/1 -> AMK FL/4(Torque_limit_neg)
  Read CM Dict2/1 -> AMK FL/1(Motor_speed_ref_in_RPM)
  AMK FL/1("Torque_output_at_wheel ") -> Eng_Torque 1/2, T_FL/1, Mux/1  "T_FL"
  Read CM Dict10/1 -> AMK FR/2(Whl_speed_rad_per_sec)
  Read CM Dict12/1 -> AMK FR/3("Torque_limit_pos ")
  Read CM Dict13/1 -> AMK FR/4(Torque_limit_neg)
  Read CM Dict24/1 -> AMK FR/1(Motor_speed_ref_in_RPM)
  AMK FR/1("Torque_Output ") -> T_FR/1, Mux/2  "T_FR"
  Read CM Dict17/1 -> AMK RL/3("Torque_limit_pos ")
  Read CM Dict18/1 -> AMK RL/4(Torque_limit_neg)
  Read CM Dict14/1 -> AMK RL/1(Motor_speed_ref_in_RPM)
  AMK RL/1("Torque_Output ") -> T_RL/1, Mux/3  "T_RL"
  Read CM Dict20/1 -> AMK RR/2(Whl_speed_rad_per_sec)
  Read CM Dict22/1 -> AMK RR/3("Torque_limit_pos ")
  Read CM Dict23/1 -> AMK RR/4(Torque_limit_neg)
  Read CM Dict19/1 -> AMK RR/1(Motor_speed_ref_in_RPM)
  AMK RR/1("Torque_Output ") -> T_RR/1, Mux/4  "T_RR"
  Mux/1 -> Gain14/1
  Gain14/1 -> "Eng_Torque "/1, To File--/1
  Read CM Dict4/1 -> Gain4/1
  Read CM Dict3/1 -> Gain6/1
  Read CM Dict5/1 -> Gain7/1
  Read CM Dict6/1 -> Gain8/1
  Read CM Dict8/1 -> Gain3/1, AMK FL/3("Torque_limit_pos ")
  Read CM Dict15/1 -> AMK RL/2(Whl_speed_rad_per_sec)
  Gain3/1 -> Eng_Torque 1/1

== system TV_2017/CarMaker/Control_System /Slip Rate Control /SMC Traction Control/Slip Rate FL ==
  SR_ref : Inport
  Kp : Inport  Port=2
  SR : Inport  Port=3
  states : Inport  Port=4
  SMC : MATLAB Function  TreatAsAtomicUnit=on
  mu lookup : Lookup_n-D  NumberOfTableDimensions=1  BreakpointsForDimension1="[0  0.15 1]"  Table=[0 1.5 0.75]  ExtrapMethod=Clip  UseLastTableValue=on  InternalRulePriority=Speed  RndMeth=Simplest  InputSameDT=on
  Tc : Outport
  wires:
  SR_ref/1 -> SMC/3(SR_ref)
  SR/1 -> SMC/2(SR), mu lookup/1
  mu lookup/1 -> SMC/1(muOfSlip)
  Kp/1 -> SMC/5(K)
  states/1 -> SMC/4(states)
  SMC/1(TC) -> Tc/1

== system TV_2017/CarMaker/Control_System /Slip Rate Control /SMC Traction Control/Slip Rate FL1 ==
  SR_ref : Inport
  Kp : Inport  Port=2
  SR : Inport  Port=3
  states : Inport  Port=4
  SMC : MATLAB Function  TreatAsAtomicUnit=on
  mu lookup : Lookup_n-D  NumberOfTableDimensions=1  BreakpointsForDimension1="[0  0.15 1]"  Table=[0 1.5 0.75]  ExtrapMethod=Clip  UseLastTableValue=on  InternalRulePriority=Speed  RndMeth=Simplest  InputSameDT=on
  Tc : Outport
  wires:
  SMC/1(TC) -> Tc/1
  states/1 -> SMC/4(states)
  Kp/1 -> SMC/5(K)
  mu lookup/1 -> SMC/1(muOfSlip)
  SR/1 -> mu lookup/1, SMC/2(SR)
  SR_ref/1 -> SMC/3(SR_ref)

== system TV_2017/CarMaker/Control_System /Slip Rate Control /SMC Traction Control/Slip Rate FL2 ==
  SR_ref : Inport
  Kp : Inport  Port=2
  SR : Inport  Port=3
  states : Inport  Port=4
  SMC : MATLAB Function  TreatAsAtomicUnit=on
  mu lookup : Lookup_n-D  NumberOfTableDimensions=1  BreakpointsForDimension1="[0  0.15 1]"  Table=[0 1.5 0.75]  ExtrapMethod=Clip  UseLastTableValue=on  InternalRulePriority=Speed  RndMeth=Simplest  InputSameDT=on
  Tc : Outport
  wires:
  SR_ref/1 -> SMC/3(SR_ref)
  SR/1 -> SMC/2(SR), mu lookup/1
  mu lookup/1 -> SMC/1(muOfSlip)
  Kp/1 -> SMC/5(K)
  states/1 -> SMC/4(states)
  SMC/1(TC) -> Tc/1

== system TV_2017/CarMaker/Control_System /Slip Rate Control /SMC Traction Control/Slip Rate FL3 ==
  SR_ref : Inport
  Kp : Inport  Port=2
  SR : Inport  Port=3
  states : Inport  Port=4
  SMC : MATLAB Function  TreatAsAtomicUnit=on
  mu lookup : Lookup_n-D  NumberOfTableDimensions=1  BreakpointsForDimension1="[0  0.15 1]"  Table=[0 1.5 0.75]  ExtrapMethod=Clip  UseLastTableValue=on  InternalRulePriority=Speed  RndMeth=Simplest  InputSameDT=on
  Tc : Outport
  wires:
  SMC/1(TC) -> Tc/1
  states/1 -> SMC/4(states)
  Kp/1 -> SMC/5(K)
  mu lookup/1 -> SMC/1(muOfSlip)
  SR/1 -> mu lookup/1, SMC/2(SR)
  SR_ref/1 -> SMC/3(SR_ref)

== system TV_2017/CarMaker/Control_System /Slip Rate Control /Traction Controllers/Slip Rate FL ==
  SR_ref : Inport
  Kp : Inport  Port=2
  Ki : Inport  Port=3
  SR : Inport  Port=4
  Ti_ref : Inport  Port=5
  Constant : Constant  Value=single(0)
  Constant1 : Constant  Value=single(0)
  Discrete-Time Integrator2 : DiscreteIntegrator  ExternalReset=either  InitialConditionSetting=State (most efficient)  SampleTime=-1  ICPrevOutput=DiscIntNeverNeededParam  ICPrevScaledInput=DiscIntNeverNeededParam
  Gain : Gain  Gain=single(-1)
  Gain1 : Gain  Gain=single(-1)
  Gain2 : Gain  Gain=tractionControl.Kb
  Gain7 : Gain  Gain=single(-1)
  Product : Product
  Product1 : Product
  Saturation Dynamic : simulink/Discontinuities/Saturation Dynamic  OutMin=[]  OutMax=[]  OutDataTypeStr=single  OutputDataTypeScalingMode=single  OutDataType=fixdt(1, 16)  OutScaling=2^-10  DoSatur=off
  Saturation Dynamic1 : simulink/Discontinuities/Saturation Dynamic  OutMin=[]  OutMax=[]  OutDataTypeStr=single  OutputDataTypeScalingMode=single  OutDataType=fixdt(1, 16)  OutScaling=2^-10  DoSatur=off
  Sum : Sum  Inputs=|+-
  Sum1 : Sum  Inputs=++|
  Sum2 : Sum  Inputs=|++
  Sum3 : Sum  Inputs=|+-  AccumDataTypeStr=single
  Switch : Switch  Criteria=u2 > Threshold
  Switch1 : Switch  Criteria=u2 > Threshold
  Switch2 : Switch  Criteria=u2 > Threshold
  TC_output : Outport
  wires:
  SR/1 -> Sum/2
  Product/1 -> Sum2/2
  Saturation Dynamic/1 -> Sum2/1, Sum3/1
  Sum/1 -> Product/2, Product1/2
  Gain1/1 -> Switch1/1
  Constant1/1 -> Switch1/3
  Constant/1 -> Switch/1
  Gain/1 -> Switch/3
  Ti_ref/1 -> Discrete-Time Integrator2/2, Switch2/2, Switch1/2, Gain1/1, Gain/1, Switch/2
  SR_ref/1 -> Gain7/1, Switch2/1
  Gain7/1 -> Switch2/3
  Switch2/1 -> Sum/1
  Switch/1 -> Saturation Dynamic1/1, Saturation Dynamic/1
  Switch1/1 -> Saturation Dynamic1/3, Saturation Dynamic/3
  Kp/1 -> Product/1
  Sum1/1 -> Discrete-Time Integrator2/1
  Ki/1 -> Product1/1
  Product1/1 -> Sum1/2
  Discrete-Time Integrator2/1 -> Saturation Dynamic/2, Sum3/2
  Sum3/1 -> Gain2/1
  Gain2/1 -> Sum1/1
  Sum2/1 -> Saturation Dynamic1/2
  Saturation Dynamic1/1 -> TC_output/1

== system TV_2017/CarMaker/Control_System /Slip Rate Control /Traction Controllers/Slip Rate FR ==
  SR_ref : Inport
  Kp : Inport  Port=2
  Ki : Inport  Port=3
  SR : Inport  Port=4
  Ti_ref : Inport  Port=5
  Constant : Constant  Value=single(0)
  Constant1 : Constant  Value=single(0)
  Discrete-Time Integrator2 : DiscreteIntegrator  ExternalReset=either  InitialConditionSetting=State (most efficient)  SampleTime=-1  ICPrevOutput=DiscIntNeverNeededParam  ICPrevScaledInput=DiscIntNeverNeededParam
  Gain : Gain  Gain=single(-1)
  Gain1 : Gain  Gain=single(-1)
  Gain2 : Gain  Gain=tractionControl.Kb
  Gain7 : Gain  Gain=single(-1)
  PI_Kp 1 : Scope
  PI_Kp 2 : Scope
  PI_Kp 4 : Scope
  Product : Product
  Product1 : Product
  Saturation Dynamic : simulink/Discontinuities/Saturation Dynamic  OutMin=[]  OutMax=[]  OutDataTypeStr=single  OutputDataTypeScalingMode=single  OutDataType=fixdt(1, 16)  OutScaling=2^-10  DoSatur=off
  Saturation Dynamic1 : simulink/Discontinuities/Saturation Dynamic  OutMin=[]  OutMax=[]  OutDataTypeStr=single  OutputDataTypeScalingMode=single  OutDataType=fixdt(1, 16)  OutScaling=2^-10  DoSatur=off
  Sum : Sum  Inputs=|+-
  Sum1 : Sum  Inputs=++|
  Sum2 : Sum  Inputs=|++
  Sum3 : Sum  Inputs=|+-  AccumDataTypeStr=single
  Switch : Switch  Criteria=u2 > Threshold
  Switch1 : Switch  Criteria=u2 > Threshold
  Switch2 : Switch  Criteria=u2 > Threshold
  integrator : Scope
  TC_output : Outport
  wires:
  Saturation Dynamic1/1 -> TC_output/1, PI_Kp 1/1
  Sum2/1 -> Saturation Dynamic1/2
  Gain2/1 -> PI_Kp 4/1, Sum1/1
  Sum3/1 -> Gain2/1
  Discrete-Time Integrator2/1 -> Sum3/2, Saturation Dynamic/2, integrator/1
  Product1/1 -> Sum1/2
  Ki/1 -> Product1/1
  Sum1/1 -> Discrete-Time Integrator2/1
  Kp/1 -> Product/1
  Switch1/1 -> Saturation Dynamic/3, Saturation Dynamic1/3
  Switch/1 -> Saturation Dynamic/1, Saturation Dynamic1/1
  Switch2/1 -> Sum/1
  Gain7/1 -> Switch2/3
  SR_ref/1 -> Switch2/1, Gain7/1
  Ti_ref/1 -> Switch2/2, Discrete-Time Integrator2/2, Switch/2, Gain/1, Gain1/1, Switch1/2
  Gain/1 -> Switch/3
  Constant/1 -> Switch/1
  Constant1/1 -> Switch1/3
  Gain1/1 -> Switch1/1
  Sum/1 -> Product1/2, Product/2
  Saturation Dynamic/1 -> Sum3/1, Sum2/1
  Product/1 -> Sum2/2, PI_Kp 2/1
  SR/1 -> Sum/2

== system TV_2017/CarMaker/Control_System /Slip Rate Control /Traction Controllers/Slip Rate RL ==
  SR_ref : Inport
  Kp : Inport  Port=2
  Ki : Inport  Port=3
  SR : Inport  Port=4
  Ti_ref : Inport  Port=5
  Constant : Constant  Value=single(0)
  Constant1 : Constant  Value=single(0)
  Discrete-Time Integrator2 : DiscreteIntegrator  ExternalReset=either  InitialConditionSetting=State (most efficient)  SampleTime=-1  ICPrevOutput=DiscIntNeverNeededParam  ICPrevScaledInput=DiscIntNeverNeededParam
  Gain : Gain  Gain=single(-1)
  Gain1 : Gain  Gain=single(-1)
  Gain2 : Gain  Gain=tractionControl.Kb
  Gain7 : Gain  Gain=single(-1)
  PI_Kp 1 : Scope
  PI_Kp 2 : Scope
  PI_Kp 4 : Scope
  Product : Product
  Product1 : Product
  Saturation Dynamic : simulink/Discontinuities/Saturation Dynamic  OutMin=[]  OutMax=[]  OutDataTypeStr=single  OutputDataTypeScalingMode=single  OutDataType=fixdt(1, 16)  OutScaling=2^-10  DoSatur=off
  Saturation Dynamic1 : simulink/Discontinuities/Saturation Dynamic  OutMin=[]  OutMax=[]  OutDataTypeStr=single  OutputDataTypeScalingMode=single  OutDataType=fixdt(1, 16)  OutScaling=2^-10  DoSatur=off
  Sum : Sum  Inputs=|+-
  Sum1 : Sum  Inputs=++|
  Sum2 : Sum  Inputs=|++
  Sum3 : Sum  Inputs=|+-  AccumDataTypeStr=single
  Switch : Switch  Criteria=u2 > Threshold
  Switch1 : Switch  Criteria=u2 > Threshold
  Switch2 : Switch  Criteria=u2 > Threshold
  integrator : Scope
  TC_output : Outport
  wires:
  Saturation Dynamic1/1 -> TC_output/1, PI_Kp 1/1
  Sum2/1 -> Saturation Dynamic1/2
  Gain2/1 -> PI_Kp 4/1, Sum1/1
  Sum3/1 -> Gain2/1
  Discrete-Time Integrator2/1 -> Sum3/2, Saturation Dynamic/2, integrator/1
  Product1/1 -> Sum1/2
  Ki/1 -> Product1/1
  Sum1/1 -> Discrete-Time Integrator2/1
  Kp/1 -> Product/1
  Switch1/1 -> Saturation Dynamic/3, Saturation Dynamic1/3
  Switch/1 -> Saturation Dynamic/1, Saturation Dynamic1/1
  Switch2/1 -> Sum/1
  Gain7/1 -> Switch2/3
  SR_ref/1 -> Switch2/1, Gain7/1
  Ti_ref/1 -> Switch2/2, Discrete-Time Integrator2/2, Switch/2, Gain/1, Gain1/1, Switch1/2
  Gain/1 -> Switch/3
  Constant/1 -> Switch/1
  Constant1/1 -> Switch1/3
  Gain1/1 -> Switch1/1
  Sum/1 -> Product1/2, Product/2
  Saturation Dynamic/1 -> Sum3/1, Sum2/1
  Product/1 -> Sum2/2, PI_Kp 2/1
  SR/1 -> Sum/2

== system TV_2017/CarMaker/Control_System /Slip Rate Control /Traction Controllers/Slip Rate RR ==
  SR_ref : Inport
  Kp : Inport  Port=2
  Ki : Inport  Port=3
  SR : Inport  Port=4
  Ti_ref : Inport  Port=5
  Constant : Constant  Value=single(0)
  Constant1 : Constant  Value=single(0)
  Discrete-Time Integrator2 : DiscreteIntegrator  ExternalReset=either  InitialConditionSetting=State (most efficient)  SampleTime=-1  ICPrevOutput=DiscIntNeverNeededParam  ICPrevScaledInput=DiscIntNeverNeededParam
  Gain : Gain  Gain=single(-1)
  Gain1 : Gain  Gain=single(-1)
  Gain2 : Gain  Gain=tractionControl.Kb
  Gain7 : Gain  Gain=single(-1)
  PI_Kp 1 : Scope
  PI_Kp 2 : Scope
  PI_Kp 4 : Scope
  Product : Product
  Product1 : Product
  Saturation Dynamic : simulink/Discontinuities/Saturation Dynamic  OutMin=[]  OutMax=[]  OutDataTypeStr=single  OutputDataTypeScalingMode=single  OutDataType=fixdt(1, 16)  OutScaling=2^-10  DoSatur=off
  Saturation Dynamic1 : simulink/Discontinuities/Saturation Dynamic  OutMin=[]  OutMax=[]  OutDataTypeStr=single  OutputDataTypeScalingMode=single  OutDataType=fixdt(1, 16)  OutScaling=2^-10  DoSatur=off
  Sum : Sum  Inputs=|+-
  Sum1 : Sum  Inputs=++|
  Sum2 : Sum  Inputs=|++
  Sum3 : Sum  Inputs=|+-  AccumDataTypeStr=single
  Switch : Switch  Criteria=u2 > Threshold
  Switch1 : Switch  Criteria=u2 > Threshold
  Switch2 : Switch  Criteria=u2 > Threshold
  integrator : Scope
  TC_output : Outport
  wires:
  SR/1 -> Sum/2
  Product/1 -> PI_Kp 2/1, Sum2/2
  Saturation Dynamic/1 -> Sum2/1, Sum3/1
  Sum/1 -> Product/2, Product1/2
  Gain1/1 -> Switch1/1
  Constant1/1 -> Switch1/3
  Constant/1 -> Switch/1
  Gain/1 -> Switch/3
  Ti_ref/1 -> Switch1/2, Gain1/1, Gain/1, Switch/2, Discrete-Time Integrator2/2, Switch2/2
  SR_ref/1 -> Gain7/1, Switch2/1
  Gain7/1 -> Switch2/3
  Switch2/1 -> Sum/1
  Switch/1 -> Saturation Dynamic1/1, Saturation Dynamic/1
  Switch1/1 -> Saturation Dynamic1/3, Saturation Dynamic/3
  Kp/1 -> Product/1
  Sum1/1 -> Discrete-Time Integrator2/1
  Ki/1 -> Product1/1
  Product1/1 -> Sum1/2
  Discrete-Time Integrator2/1 -> integrator/1, Saturation Dynamic/2, Sum3/2
  Sum3/1 -> Gain2/1
  Gain2/1 -> Sum1/1, PI_Kp 4/1
  Sum2/1 -> Saturation Dynamic1/2
  Saturation Dynamic1/1 -> PI_Kp 1/1, TC_output/1

== system TV_2017/CarMaker/Control_System /Subsystem/2016 adapted/Torque Allocation ==
  T_req : Inport
  states : Inport  Port=2
  maxMotorTorque : Inport  Port=3
  Mz_ref : Inport  Port=4
  Mux1 : Mux  Inputs=3
  Mz : Scope
  Ti_max : Scope
  TorqueAllocation : MATLAB Function  TreatAsAtomicUnit=on
  Ti_lim : Outport
  Mz_allocated : Outport  Port=2
  wires:
  T_req/1 -> TorqueAllocation/1(T_req)
  states/1 -> TorqueAllocation/2(states)
  TorqueAllocation/1(Ti_lim) -> Ti_lim/1
  Mz_ref/1 -> Mux1/3, TorqueAllocation/4(Mz_ref)  "Mz_ref"
  TorqueAllocation/2(Ti_max) -> Ti_max/1
  TorqueAllocation/3(Mz_error) -> Mux1/1  "Mz_error"
  TorqueAllocation/4(Mz_allocated) -> Mux1/2, Mz_allocated/1  "Mz_all"
  Mux1/1 -> Mz/1
  maxMotorTorque/1 -> TorqueAllocation/3(maxMotorTorque)

== system TV_2017/CarMaker/Control_System /Subsystem/Torque allocation 2016/Torque Allocation ==
  T_req : Inport
  states : Inport  Port=2
  maxMotorTorque : Inport  Port=3
  Mz_ref : Inport  Port=4
  Mux1 : Mux  Inputs=3
  Mz : Scope
  Ti_max : Scope
  TorqueAllocation : MATLAB Function  TreatAsAtomicUnit=on
  Ti_lim : Outport
  Mz_error : Outport  Port=2
  wires:
  T_req/1 -> TorqueAllocation/1(T_req)
  states/1 -> TorqueAllocation/2(states)
  TorqueAllocation/1(Ti_lim) -> Ti_lim/1
  Mz_ref/1 -> Mux1/3, TorqueAllocation/4(Mz_ref)  "Mz_ref"
  TorqueAllocation/2(Ti_max) -> Ti_max/1
  TorqueAllocation/3(Mz_error) -> Mux1/1, Mz_error/1  "Mz_error"
  TorqueAllocation/4(Mz_allocated) -> Mux1/2  "Mz_all"
  Mux1/1 -> Mz/1
  maxMotorTorque/1 -> TorqueAllocation/3(maxMotorTorque)

== system TV_2017/CarMaker/Estimations/Fz_estimators/Fz_Estimation/1st_deriv ==
  signal : Inport
  delta_t : Inport  Port=2
  Diff_Function : MATLAB Function  TreatAsAtomicUnit=on
  Memory : Memory  X0=[0;0;0;0;0;0;0;0;0;0;0;0;0;0;0]
  deriv : Outport
  wires:
  delta_t/1 -> Diff_Function/3(delta_t)
  Diff_Function/2(y) -> deriv/1
  signal/1 -> Diff_Function/2(sig)
  Diff_Function/1(y_old) -> Memory/1
  Memory/1 -> Diff_Function/1("y_old ")

== system TV_2017/CarMaker/Estimations/Fz_estimators/Fz_Estimation/2nd_deriv ==
  signal : Inport
  delta_t : Inport  Port=2
  Diff_Function : MATLAB Function  TreatAsAtomicUnit=on
  Memory : Memory  X0=[0;0;0;0;0;0;0;0;0;0]
  deriv : Outport
  wires:
  delta_t/1 -> Diff_Function/3(delta_t)
  Diff_Function/2(y) -> deriv/1
  signal/1 -> Diff_Function/2(sig)
  Diff_Function/1(y_old) -> Memory/1
  Memory/1 -> Diff_Function/1("y_old ")

== system TV_2017/CarMaker/IPG Vehicle3/CarAndTrailer/CarAndTrailerUpd/CreateBus Brake.IF.In ==
  In : Inport
  BusCreator : BusCreator  Inputs=9
  Demux : Demux  Outputs=9
  Out : Outport
  wires:
  Demux/9 -> BusCreator/9  "Brake IF Trq_Reg RR"
  Demux/8 -> BusCreator/8  "Brake IF Trq_Reg RL"
  Demux/7 -> BusCreator/7  "Brake IF Trq_Reg FR"
  Demux/6 -> BusCreator/6  "Brake IF Trq_Reg FL"
  Demux/5 -> BusCreator/5  "Brake IF Trq_Reg_max RR"
  Demux/4 -> BusCreator/4  "Brake IF Trq_Reg_max RL"
  Demux/3 -> BusCreator/3  "Brake IF Trq_Reg_max FR"
  Demux/2 -> BusCreator/2  "Brake IF Trq_Reg_max FL"
  Demux/1 -> BusCreator/1  "Brake IF T_env"
  BusCreator/1 -> Out/1
  In/1 -> Demux/1

== system TV_2017/CarMaker/IPG Vehicle3/CarAndTrailer/Forces/External Suspension Forces ==
  note: The FSpring/FDamp/FStabi/FBuf outputs of this subsystem will be
      | active if the SuspExtFrcs.Kind entry in the vehicle parameter file
      | is either not present or is empty or has the value "CM4SL".
  note: Insert your suspension forces model here.
  Sync_In : Inport
  lSpring : Inport  Port=2
  vDamp : Inport  Port=3
  lStabi : Inport  Port=4
  lBuf : Inport  Port=5
  Bus Creator{,5..7} (4 alike) : BusCreator  Inputs=8
  Bus Creator{1..4} (4 alike) : BusCreator  Inputs=4
  Demux{1..4} (4 alike) : Demux  Outputs=8
  Ground{,1..15} (16 alike) : Ground
  Terminator{1..4,12} (5 alike) : Terminator
  FSpring : Outport
  FDamp : Outport  Port=2
  FStabi : Outport  Port=3
  FBuf : Outport  Port=4
  wires:
  Bus Creator7/1 -> Terminator4/1
  Bus Creator6/1 -> Terminator3/1
  Bus Creator5/1 -> Terminator2/1
  Bus Creator/1 -> Terminator1/1
  Demux4/8 -> Bus Creator7/8  "vBuf RR"
  Demux4/7 -> Bus Creator7/7  "vBuf RL"
  Demux4/6 -> Bus Creator7/6  "vBuf FR"
  Demux4/5 -> Bus Creator7/5  "vBuf FL"
  Demux3/8 -> Bus Creator6/8  "vStabi RR"
  Demux3/7 -> Bus Creator6/7  "vStabi RL"
  Demux3/6 -> Bus Creator6/6  "vStabi FR"
  Demux3/5 -> Bus Creator6/5  "vStabi FL"
  Demux2/8 -> Bus Creator5/8  "vDamp RR"
  Demux2/7 -> Bus Creator5/7  "vDamp RL"
  Demux2/6 -> Bus Creator5/6  "vDamp FR"
  Demux2/5 -> Bus Creator5/5  "vDamp FL"
  Demux1/8 -> Bus Creator/8  "vSpring RR"
  Demux1/7 -> Bus Creator/7  "vSpring RL"
  Demux1/6 -> Bus Creator/6  "vSpring FR"
  Demux1/5 -> Bus Creator/5  "vSpring FL"
  Demux2/4 -> Bus Creator5/4  "lDamp RR"
  Demux2/3 -> Bus Creator5/3  "lDamp RL"
  Demux2/2 -> Bus Creator5/2  "lDamp FR"
  Demux2/1 -> Bus Creator5/1  "lDamp FL"
  Demux1/4 -> Bus Creator/4  "lSpring RR"
  Demux1/3 -> Bus Creator/3  "lSpring RL"
  Demux1/2 -> Bus Creator/2  "lSpring FR"
  Demux1/1 -> Bus Creator/1  "lSpring FL"
  Demux3/4 -> Bus Creator6/4  "lStabi RR"
  Demux3/3 -> Bus Creator6/3  "lStabi RL"
  Demux3/2 -> Bus Creator6/2  "lStabi FR"
  Demux3/1 -> Bus Creator6/1  "lStabi FL"
  lStabi/1 -> Demux3/1
  vDamp/1 -> Demux2/1
  lSpring/1 -> Demux1/1
  Demux4/4 -> Bus Creator7/4  "lBuf RR"
  Demux4/3 -> Bus Creator7/3  "lBuf RL"
  Demux4/2 -> Bus Creator7/2  "lBuf FR"
  Demux4/1 -> Bus Creator7/1  "lBuf FL"
  lBuf/1 -> Demux4/1
  Ground14/1 -> Bus Creator4/1  "FBuf FL"
  Ground15/1 -> Bus Creator4/2  "FBuf FR"
  Ground12/1 -> Bus Creator4/3  "FBuf RL"
  Ground13/1 -> Bus Creator4/4  "FBuf RR"
  Bus Creator4/1 -> FBuf/1
  Sync_In/1 -> Terminator12/1
  Bus Creator2/1 -> FSpring/1
  Ground/1 -> Bus Creator2/1  "FSpring FL"
  Ground1/1 -> Bus Creator2/2  "FSpring FR"
  Ground2/1 -> Bus Creator2/3  "FSpring RL"
  Ground3/1 -> Bus Creator2/4  "FSpring RR"
  Ground4/1 -> Bus Creator1/1  "FDamp FL"
  Ground5/1 -> Bus Creator1/2  "FDamp FR"
  Ground6/1 -> Bus Creator1/3  "FDamp RL"
  Ground7/1 -> Bus Creator1/4  "FDamp RR"
  Bus Creator1/1 -> FDamp/1
  Ground8/1 -> Bus Creator3/1  "FStabi FL"
  Ground9/1 -> Bus Creator3/2  "FStabi FR"
  Ground10/1 -> Bus Creator3/3  "FStabi RL"
  Ground11/1 -> Bus Creator3/4  "FStabi RR"
  Bus Creator3/1 -> FStabi/1
